simulink model "control_constraint"  (R2024a)
settings: Solver=VariableStepAuto  StartTime=0.0  StopTime=5  RelTol=1e-3
values from neighbouring files (symbols this model uses):
  lbz = 0.4    [init.m]
  params = [m1; m2; a1; a2; kj1; kj2; lbz-rj1; ac1; ac2]    [init_mpc.m]    (also in init_mpc_EKF.m; init_mpc_constraint.m; stateFcnRoboticArmEKF.m = uk(3:11))
  rect_lx = 0.2    [init_mpc_constraint.m]
  rect_ly = 0.2    [init_mpc_constraint.m]
  rect_lz = 0.5    [init_mpc_constraint.m]
  rect_xcenter = 0.15    [init_mpc_constraint.m]
  rect_ycenter = 0.2    [init_mpc_constraint.m]
  rect_zcenter = 0.25    [init_mpc_constraint.m]
undefined symbols (not defined in the file or in its folder): X, Y, Z
libraries: sm_lib x4, mpclib x1, SignalEditorBlockLib x1, nesl_utility x1
settings Model: Creator=berto  LastModifiedBy=berto

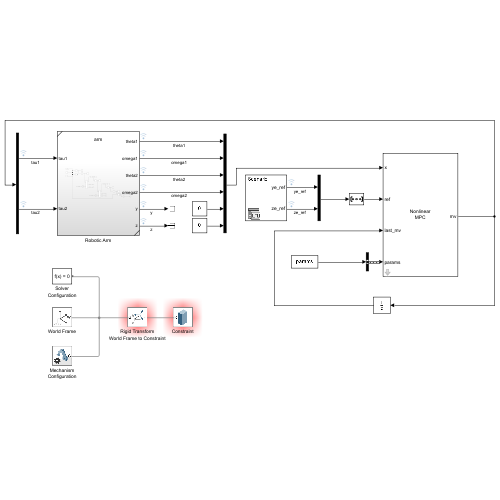
[thumbnail: Simulink's stored preview of the top-level diagram]
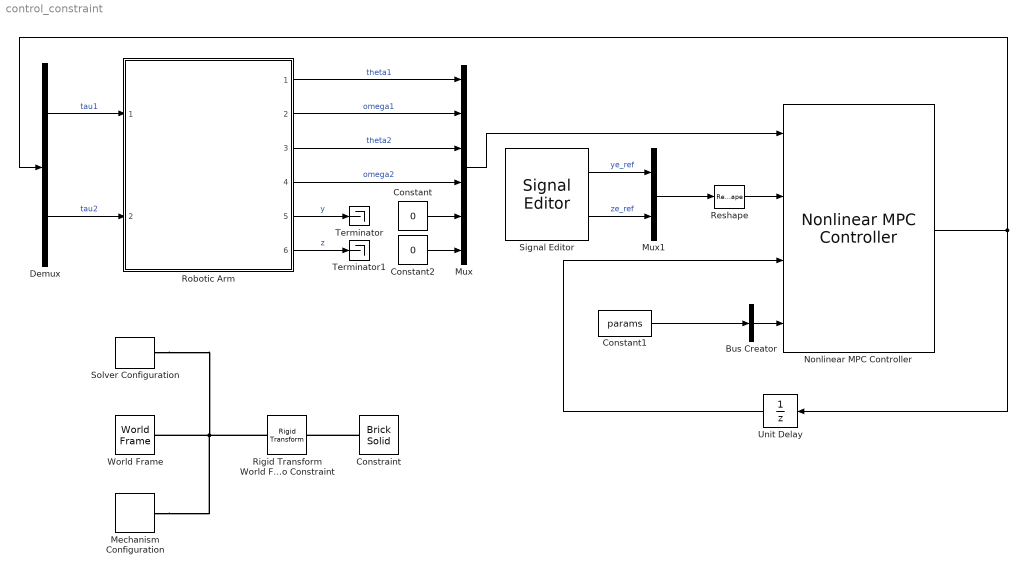
== system control_constraint ==
  Bus Creator : BusCreator  Inputs=1  OutDataTypeStr=Bus: paramsBusObject  NonVirtualBus=on
      settings: InheritFromInputs=off
  Constant : Constant  Value=0
  Constant1 : Constant  Value=params
  Constant2 : Constant  Value=0
  Constraint : sm_lib/Body Elements/Brick Solid  BrickDimensions=[rect_lx rect_ly rect_lz]  BrickDimensionsUnits=m  ExportEntireGeometry=off  InertiaType=CalculateFromGeometry  BasedOnType=Density  Density=rho_steel  DensityUnits=kg/m^3  Mass=1  MassUnits=kg  CenterOfMass=[0 0 0]  CenterOfMassUnits=m  MomentsOfInertia=[1 1 1]  MomentsOfInertiaUnits=kg*m^2  ProductsOfInertia=[0 0 0]  ProductsOfInertiaUnits=kg*m^2  GraphicType=FromGeometry  MarkerShape=Sphere  MarkerSize=10  GraphicVisPropType=SimpleVisualProperties  GraphicDiffuseColor=[0.5 0.5 0.5]  GraphicOpacity=1  GraphicSpecularColor=[0.5 0.5 0.5 1.0]  GraphicAmbientColor=[0.15 0.15 0.15 1.0]  GraphicEmissiveColor=[0.0 0.0 0.0 1.0]  GraphicShininess=75  DoExposeReferenceFrame=on  SerializedFrames=<Frames/>
  Demux : Demux  Outputs=2
  Mechanism Configuration : sm_lib/Utilities/Mechanism Configuration  UniformGravity=Constant  GravityVector=[0 0 -9.80665]  GravityVectorUnits=m/s^2  LinearizationDelta=0.001  JointModeTransitionNonlinearIterations=2
  Mux : Mux  Inputs=6
  Mux1 : Mux  Inputs=2
  Nonlinear MPC Controller : mpclib/Nonlinear MPC Controller  nlmpcobj=nlobj  UseObjectTs=on  UseMEX=off  md_enabled=off  mvtarget_enabled=off  param_enabled=on  cost_enabled=off  mvseq_enabled=off  stateseq_enabled=off  ovseq_enabled=off  slack_enabled=off  status_enabled=off  ov_min=off  ov_max=off  mv_min=off  mv_max=off  mvrate_min=off  mvrate_max=off  state_min=off  state_max=off  ov_weight=off  mv_weight=off  mvrate_weight=off  ecr_weight=off  nlp_initialize=off
  Reshape : Reshape  OutputDimensionality=Row vector (2-D)
  Rigid Transform World Frame to Constraint : sm_lib/Frames and Transforms/Rigid Transform  RotationMethod=None  FollAlignAxisA=+X  BaseAlignAxisA=+Y  FollAlignAxisB=+Y  BaseAlignAxisB=+Z  RotationStandardAxis=+Y  RotationAngle=0  RotationAngleUnits=deg  RotationArbitraryAxis=[0 0 1]  RotationSequenceAxes=FollowerAxes  RotationSequence=XYX  RotationSequenceAngles=[0 0 0]  RotationSequenceAnglesUnits=deg  RotationMatrix=[1 0 0;0 1 0;0 0 1]  Quaternion=[1 0 0 0]  TranslationMethod=Cartesian  TranslationCartesianOffset=[rect_xcenter rect_ycenter rect_zcenter]  TranslationCartesianOffsetUnits=m  TranslationStandardAxis=+Z  TranslationStandardOffset=lbz/2  TranslationStandardOffsetUnits=m  TranslationROffset=0  TranslationROffsetUnits=m  TranslationThetaOffset=0  TranslationThetaOffsetUnits=deg  TranslationZOffset=0  TranslationZOffsetUnits=m
  Robotic Arm : Subsystem  ReferencedSubsystem=arm
  Signal Editor : SignalEditorBlockLib/Signal Editor  FileName=ref.mat  ActiveScenario=Scenario1  ActiveSignal=ye_ref  IsBus=off  OutputBusObjectStr=Bus: BusObject  SampleTime=0  Interpolate=off  ZeroCross=off  OutputAfterFinalValue=Setting to zero  Unit=inherit  PreserveSignalName=on  ApplySigPropsToAllScenarios=on  ApplySigPropsToAllSignals=off
  Solver Configuration : nesl_utility/Solver Configuration  PhysicalDomain=network_engine_domain  SubClassName=solver  LeftPortType=input  RightPortType=generic  Tones=[]  Harmonics=[]  SimulateNoise=off  Profile=off  UseLocalSampling=off  EnableSwitchedLinearOptims=on  FrequencyDomain=off  UseCCode=off  RelTol=0.001  AbsTol=1e-06  MinStep=1e-09  ToWorkspace=off  RevertToSquareIcSolve=off  NumHomotopyIterations=100  PhasorMode=off  PhasorModeNumHarmonics=1  ConsistencySolver=NEWTON_XTOL_AFTER_FTOL  IndexReductionMethod=DerivativeReplacement  DoDC=off  ResidualTolerance=1e-09  ConsistencyTolSource=GLOBAL  ConsistencyAbsTol=0.001  ConsistencyRelTol=0.001  ConsistencyTolFactor=0.001  UseLocalSolver=off  LocalSolverChoice=NE_BACKWARD_EULER_ADVANCER  ResolveIndetEquations=on  FunctionEvalNumThread=1  LocalSolverSampleTime=0.001  DoFixedCost=off  MaxNonlinIter=3  MaxModeIter=2  ComputeImpulses=off  ImpulseIterations=2  LinearAlgebra=Sparse  LinearAlgebraNumThread=0  EquationFormulation=NE_TIME_EF  DelaysMemoryBudget=1024  AutomaticFiltering=on  FilteringTimeConstant=0.1  PartitionStorageMethod=AS_NEEDED  PartitionMemoryBudget=1024  PartitionMethod=FAST  MultibodyUseLocalSolver=off  MultibodyLocalSolverChoice=ODE1  MultibodyLocalSolverSampleTime=0.001
  Terminator : Terminator
  Terminator1 : Terminator
  Unit Delay : UnitDelay  SampleTime=-1  HasFrameUpgradeWarning=on
  World Frame : sm_lib/Frames and Transforms/World Frame
  wires:
  Robotic Arm/1 -> Mux/1  "theta1"
  Robotic Arm/3 -> Mux/3  "theta2"
  Robotic Arm/2 -> Mux/2  "omega1"
  Robotic Arm/4 -> Mux/4  "omega2"
  Mux/1 -> Nonlinear MPC Controller/1
  Nonlinear MPC Controller/1 -> Unit Delay/1, Demux/1
  Unit Delay/1 -> Nonlinear MPC Controller/3
  Demux/1 -> Robotic Arm/1  "tau1"
  Demux/2 -> Robotic Arm/2  "tau2"
  Constant1/1 -> Bus Creator/1
  Bus Creator/1 -> Nonlinear MPC Controller/4
  Reshape/1 -> Nonlinear MPC Controller/2
  Robotic Arm/5 -> Terminator/1  "y"
  Robotic Arm/6 -> Terminator1/1  "z"
  Signal Editor/1 -> Mux1/1  "ye_ref"
  Signal Editor/2 -> Mux1/2  "ze_ref"
  Mux1/1 -> Reshape/1
  Constant/1 -> Mux/5
  Constant2/1 -> Mux/6
  connections:
  Constraint/RConn1 -- Rigid Transform World Frame to Constraint/RConn1
  Rigid Transform World Frame to Constraint/LConn1 -- Mechanism Configuration/RConn1 -- Solver Configuration/RConn1 -- World Frame/RConn1
